simulink model "mfordmodel_v1"  (R2023a)
settings: Solver=ode45  StartTime=0.0  StopTime=10.0  RelTol=1e-3  EnableMultiTasking=on
undefined symbols (not defined in the file): ABV_RATIO_SW, AC_OFF_DLY, ACLOD, AUTO_TRNS_SW, BRAKE_DNDT_X, BZZRPM, BZZRPM_ALT, BZZTM, BZZTM_ALT, CMD_LITOFF, CMD_STABLE, CO_ST_ECT__A, COOL_BASE, DAS_BKDLY_A, DAS_CNT, DAS_CTDLY, DAS_LC_SW__A, DASCLP_5INH, DASCTL, DASMHYST, DASMPH, DEBYCP, DES_BASE, DPNEU_MUL, DSDRPM_DN_TC, DSDRPM_OFF, DSDRPM_UP_TC, EDF_DELAY, EDFHP, ETC_CL_TP, ETC_HP, GR_CM_CREEP, HCAM_ACT_CLP, HEDFHP, HEDFRPM, HICAM_PS, IAC_CAL_SW, IAC_ER_TM1, IAC_ER_TM2, IAC_ER_TM4, IAC_HI_LIM__A, IAC_ISFL_OBD, IAC_KAM_SW, IAC_LO_LIM__A, IAC_MON_TM, IAC_OT_REQ, IAC_RUN_TM, IAC_TP_OBD, IAC_TR_DAS, IAC_TST_DC, ID_DAS__A, ID_NOVS__A, IDVS_CH__A, IDVS_SL__A, IPSI_SW, IPSIDLY, IS_DRBASE__A, IS_DRBASE_A__A, IS_NUBASE__A, IS_NUBASE_A__A ... (+35)
libraries: simulink x2
(part 3 of 12)

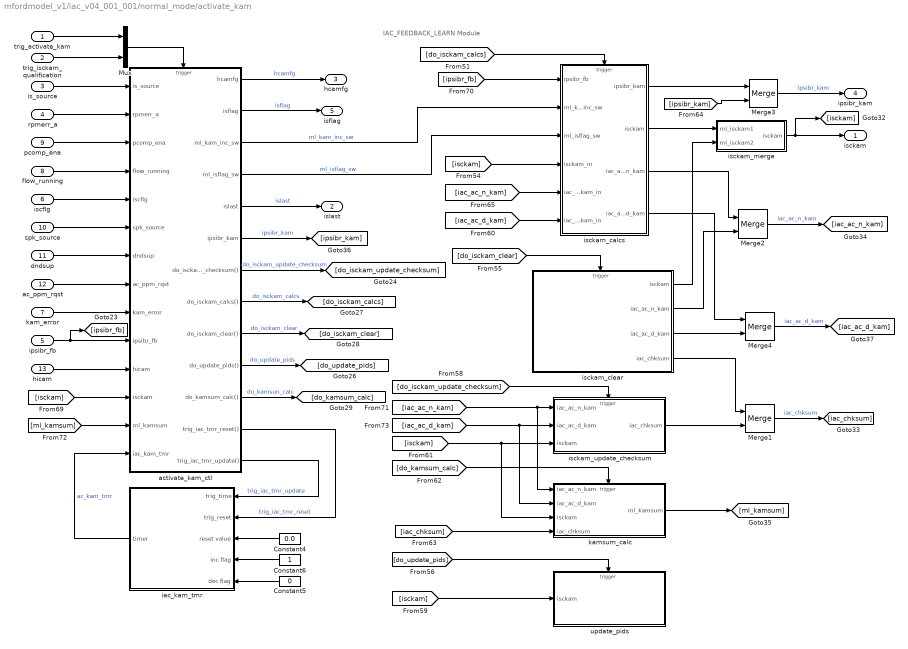
== system mfordmodel_v1/iac_v04_001_001/normal_mode/activate_kam ==
  note: IAC_FEEDBACK_LEARN Module
  trig_activate_kam : Inport
  trig_isckam_qualification : Inport  Port=2
  is_source : Inport  Port=3
  rpmerr_a : Inport  Port=4
  ipsibr_fb : Inport  Port=5
  iscflg : Inport  Port=6
  kam_error : Inport  Port=7
  flow_running : Inport  Port=8
  pcomp_ena : Inport  Port=9
  spk_source : Inport  Port=10
  dndsup : Inport  Port=11
  ac_ppm_rqst : Inport  Port=12
  hicam : Inport  Port=13
  Constant4 : Constant  Value=0.0
  Constant5 : Constant  Value=0
  Constant6 : Constant
  Merge{1..4} (4 alike) : Merge
  Mux : Mux  Inputs=2
  activate_kam_ctl : Stateflow chart  TreatAsAtomicUnit=on
  iac_kam_tmr : Subsystem  mask(TIMER){timer_name=iac_kam_tmr, init_value=0, clipped=off, tmin=, tmax=, unit_str=seconds}
      mask prompts: timer_name "Enter Timer Name"; init_value "initial TIMER value (in seconds)"; clipped "Clip timer?"; tmin "Minimum clip"; tmax "Maximum clip"; unit_str "Select timer units"
      mask help: Acts as a timer. Can count up, down, hold, or reset to zero. The required inputs are a timer function call, a reset function call, a reset value, an increment flag, and a decrement flag. Timer initial value, max and min clip values and timer name are selected below.
      mask init: same as mfordmodel_v1/iac_v04_001_001/normal_mode/activate_feedforward/ac_ppm_tmr
      mask Help:
      | <b><font size="+2">Input/Output Ports</font></b><br>
      | <p>
      | <b>Trig_timer:</b><br>
      | Connect a function call input to the 'trig_timer' port.  A function call passed through this port will activate the TIMER tool.  Activation updates the TIMER output.
      | <p>
      | <b>Trig_reset:</b><br>
      | Connect a function call input to the 'trig_reset' port.  A function call passed through this port will activate the TIMER tool.  Activation resets the TIMER output to the value passed to the 'reset_value' port.
      | <p>
      | <b>Reset_value:</b><br>
      | When 'trig_reset' is activated, the TIMER value will be reset to the real value passed to this input.
      | <p>
      | <b>Increment_flag and decrement_flag:</b><br>
      | If 'increment_flag' is 1 and 'decrement_flag' is 0, TIMER counts up.
      | If 'decrement_flag' is 1 and 'increment_flag' is 0, TIMER counts down.
      | If the flags are both 0 or both 1, TIMER holds its current value.
      | <p>
      | <b><font size="+2">Parameter Selection:</font></b>
      | <p>
      | <b>Initial TIMER Value:</b><br>
      | TIMER will begin at specified value.  Enter in seconds.
      mask TypeOptions unit_str: seconds | milliseconds
      mask Display:
      | plot( [0.3 0.45 0.55 0.7], [0.4 0.4 0.6 0.6])
      | plot( [ .475 .435 .415  .4 .4  .415 .435 .475  .525 .565 .585 .6 .6  ...
      | .585 .565 .525 .475], [.9  .885 .865  .825 .775 .735 .715  .7 .7 ...
      | .715 .735 .775 .825  .865 .885 .9 .9] )
      | plot( [.5 .5], [.89 .87])
      | plot( [.5 .5], [.71 .73])
      | plot( [.41 .43], [.8 .8])
      | plot( [.57 .59], [.8 .8])
      | plot( [.5 .5], [.8 .89])
      | plot( [.49 .5 .51], [.88 .89 .88] )
      | plot( [.5 .555], [.8 .825] )
      | plot( [.535 .555 .555], [.825 .825 .815])
      | text(0.35, 0.35, min_text)
      | text(0.6, 0.7,max_text)
      | text( 0.35, .95, timer_name)
  isckam_calcs : Subsystem  TreatAsAtomicUnit=on
  isckam_clear : Subsystem  TreatAsAtomicUnit=on  mask(isckam_clear){}
      mask help: TBD
      mask Display:
      | disp('
      | isckam0 = IAC_DR_START               \n
      | isckam1 = 0.0                                  \n
      | isckam2 = IAC_NU_START               \n
      | isckam3 = 0.0                                  \n
      | iac_ac_d_kam = IAC_AC_START       \n
      | iac_ac_n_kam = IAC_AC_START       \n
      | iac_chksum = ( isckam2 + isckam0 + \n
      |  iac_ac_d_kam + iac_ac_n_kam)         ' )
  isckam_merge : Subsystem  mask(vector_merge){}
      mask help: Merge the four elements of the "isckam" vector.
      mask Display: disp('Merge( isckam[i] )')
  isckam_update_checksum : Subsystem  TreatAsAtomicUnit=on  mask(isckam_update_checksum){}
      mask help: Computes and returns the checksum.
      mask Display:
      | disp('
      | iac_chksum = isckam[0] + \n
      |  isckam[2] +          \n
      | iac_ac_d_kam +  \n
      | iac_ac_n_ham     ')
  kamsum_calc : Subsystem  TreatAsAtomicUnit=on  mask(kam_sum_calc){}
      mask help: TBD
      mask Display:
      | fprintf(' ml_kamsum = ABS ( isckam[0] + \n
      | isckam[2] + iac_ac_n_kam + \n
      | iac_ac_d_kam - iac_chksum )')
  update_pids : Subsystem  TreatAsAtomicUnit=on  mask(update_pids){}
      mask help: Update isckam PIDS.
      mask Display:
      | disp ('Update the following PIDS:\n
      | J2190_0x0976 = isckam[0]\n
      | J2190_0x0977 = isckam[1]\n
      | J2190_0x0978 = isckam[2]\n
      | J2190_0x0979 = isckam[3]')
  isckam : Outport  InitialOutput=0
  islast : Outport  Port=2  InitialOutput=0
  hcamfg : Outport  Port=3  InitialOutput=0
  ipsibr_kam : Outport  Port=4  InitialOutput=0
  isflag : Outport  Port=5  InitialOutput=0
  wires:
  rpmerr_a/1 -> activate_kam_ctl/2(rpmerr_a)
  is_source/1 -> activate_kam_ctl/1(is_source)
  pcomp_ena/1 -> activate_kam_ctl/3(pcomp_ena)
  flow_running/1 -> activate_kam_ctl/4(flow_running)
  iscflg/1 -> activate_kam_ctl/5(iscflg)
  spk_source/1 -> activate_kam_ctl/6(spk_source)
  dndsup/1 -> activate_kam_ctl/7(dndsup)
  ac_ppm_rqst/1 -> activate_kam_ctl/8(ac_ppm_rqst)
  kam_error/1 -> activate_kam_ctl/9(kam_error)
  activate_kam_ctl/1(hcamfg) -> hcamfg/1  "hcamfg"
  activate_kam_ctl/5(islast) -> islast/1  "islast"
  [isckam] -> activate_kam_ctl/12(isckam)
  activate_kam_ctl/7(do_isckam_update_checksum()) -> [do_isckam_update_checksum]  "do_isckam_update_checksum"
  activate_kam_ctl/10(do_update_pids()) -> [do_update_pids]  "do_update_pids"
  activate_kam_ctl/12(trig_iac_tmr_reset()) -> iac_kam_tmr/2(trig_reset)  "trig_iac_tmr_reset"
  activate_kam_ctl/13(trig_iac_tmr_update()) -> iac_kam_tmr/1(trig_time)  "trig_iac_tmr_update"
  Constant5/1 -> iac_kam_tmr/5(dec flag)
  activate_kam_ctl/8(do_isckam_calcs()) -> [do_isckam_calcs]  "do_isckam_calcs"
  activate_kam_ctl/9(do_isckam_clear()) -> [do_isckam_clear]  "do_isckam_clear"
  hicam/1 -> activate_kam_ctl/11(hicam)
  trig_activate_kam/1 -> Mux/1
  Mux/1 -> activate_kam_ctl/Trigger
  trig_isckam_qualification/1 -> Mux/2
  activate_kam_ctl/11(do_kamsum_calc()) -> [do_kamsum_calc]  "do_kamsun_calc"
  Constant6/1 -> iac_kam_tmr/4(inc flag)
  Constant4/1 -> iac_kam_tmr/3(reset value)
  iac_kam_tmr/1(timer) -> activate_kam_ctl/14(iac_kam_tmr)  "ac_kam_tmr"
  [ml_kamsum] -> activate_kam_ctl/13(ml_kamsum)
  activate_kam_ctl/6(ipsibr_kam) -> [ipsibr_kam]  "ipsibr_kam"
  activate_kam_ctl/2(isflag) -> isflag/1  "isflag"
  isckam_clear/4(iac_chksum) -> Merge1/1
  [do_isckam_clear] -> isckam_clear/Trigger
  isckam_clear/1(isckam) -> isckam_merge/2(ml_isckam2)
  isckam_calcs/2(isckam) -> isckam_merge/1(ml_isckam1)
  isckam_calcs/3(iac_ac_n_kam) -> Merge2/1
  activate_kam_ctl/3(ml_kam_inc_sw) -> isckam_calcs/2(ml_kam_inc_sw)  "ml_kam_inc_sw"
  activate_kam_ctl/4(ml_isflag_sw) -> isckam_calcs/3(ml_isflag_sw)  "ml_isflag_sw"
  [do_isckam_calcs] -> isckam_calcs/Trigger
  [ipsibr_fb] -> isckam_calcs/1(ipsibr_fb)
  [isckam] -> isckam_calcs/4(isckam_in)
  [iac_ac_d_kam] -> isckam_calcs/6(iac_ac_d_kam_in)
  isckam_calcs/1(ipsibr_kam) -> Merge3/1
  [ipsibr_kam] -> Merge3/2
  Merge3/1 -> ipsibr_kam/1  "ipsibr_kam"
  isckam_calcs/4(iac_ac_d_kam) -> Merge4/1
  [iac_ac_n_kam] -> isckam_calcs/5(iac_ac_n_kam_in)
  isckam_clear/2(iac_ac_n_kam) -> Merge2/2
  isckam_clear/3(iac_ac_d_kam) -> Merge4/2
  isckam_merge/1(isckam) -> isckam/1, [isckam]
  [do_isckam_update_checksum] -> isckam_update_checksum/Trigger
  [isckam] -> update_pids/1(isckam)
  [do_update_pids] -> update_pids/Trigger
  isckam_update_checksum/1(iac_chksum) -> Merge1/2
  kamsum_calc/1(ml_kamsum) -> [ml_kamsum]
  [do_kamsum_calc] -> kamsum_calc/Trigger
  [iac_ac_n_kam] -> isckam_update_checksum/1(iac_ac_n_kam), kamsum_calc/1(iac_ac_n_kam)
  [isckam] -> isckam_update_checksum/3(isckam), kamsum_calc/3(isckam)
  [iac_chksum] -> kamsum_calc/4(iac_chksum)
  [iac_ac_d_kam] -> isckam_update_checksum/2(iac_ac_d_kam), kamsum_calc/2(iac_ac_d_kam)
  Merge2/1 -> [iac_ac_n_kam]  "iac_ac_n_kam"
  Merge1/1 -> [iac_chksum]  "iac_chksum"
  Merge4/1 -> [iac_ac_d_kam]  "iac_ac_d_kam"
  ipsibr_fb/1 -> [ipsibr_fb], activate_kam_ctl/10(ipsibr_fb)

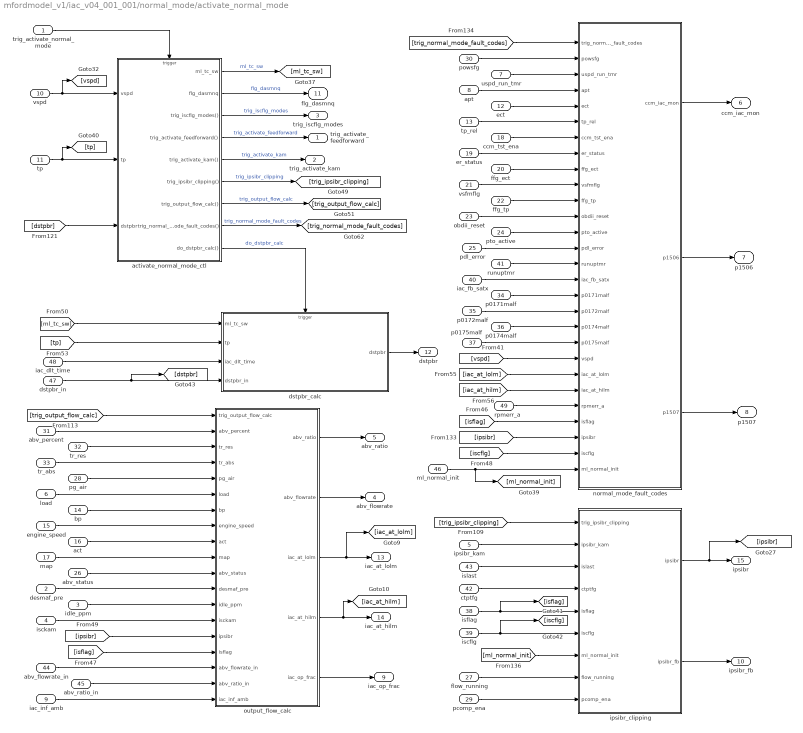
== system mfordmodel_v1/iac_v04_001_001/normal_mode/activate_normal_mode ==
  trig_activate_normal_mode : Inport
  desmaf_pre : Inport  Port=2
  idle_ppm : Inport  Port=3
  isckam : Inport  Port=4
  ipsibr_kam : Inport  Port=5
  load : Inport  Port=6
  uspd_run_tmr : Inport  Port=7
  apt : Inport  Port=8
  iac_inf_amb : Inport  Port=9
  vspd : Inport  Port=10
  tp : Inport  Port=11
  ect : Inport  Port=12
  tp_rel : Inport  Port=13
  bp : Inport  Port=14
  engine_speed : Inport  Port=15
  act : Inport  Port=16
  map : Inport  Port=17
  ccm_tst_ena : Inport  Port=18
  er_status : Inport  Port=19
  ffg_ect : Inport  Port=20
  vsfmflg : Inport  Port=21
  ffg_tp : Inport  Port=22
  obdii_reset : Inport  Port=23
  pto_active : Inport  Port=24
  pdl_error : Inport  Port=25
  abv_status : Inport  Port=26
  flow_running : Inport  Port=27
  pg_air : Inport  Port=28
  pcomp_ena : Inport  Port=29
  powsfg : Inport  Port=30
  abv_percent : Inport  Port=31
  tr_res : Inport  Port=32
  tr_abs : Inport  Port=33
  p0171malf : Inport  Port=34
  p0172malf : Inport  Port=35
  p0174malf : Inport  Port=36
  p0175malf : Inport  Port=37
  isflag : Inport  Port=38
  iscflg : Inport  Port=39
  iac_fb_satx : Inport  Port=40
  runuptmr : Inport  Port=41
  ctptfg : Inport  Port=42
  islast : Inport  Port=43
  abv_flowrate_in : Inport  Port=44
  abv_ratio_in : Inport  Port=45
  ml_normal_init : Inport  Port=46
  dstpbr_in : Inport  Port=47
  iac_dlt_time : Inport  Port=48
  rpmerr_a : Inport  Port=49
  activate_normal_mode_ctl : Stateflow chart  TreatAsAtomicUnit=on
  dstpbr_calc : Subsystem  TreatAsAtomicUnit=on  mask(dstpbr_calc){}
      mask help: TBD
      mask Display:
      | disp('\n
      | IF (ml_tc_sw == 1) THEN                                      \n
      | Tau = TCDASU                                              \n
      | ELSE IF (ml_tc_sw == 2) THEN                            \n
      | Tau = TCDASD                                              \n
      | ENDIF                                                                  \n
      | dstpbr = rolav_tc(dstpbr_in, tp, iac_dlt_time, Tau)     \n\n
      | ')
  ipsibr_clipping : Subsystem
  normal_mode_fault_codes : Subsystem
  output_flow_calc : Subsystem
  trig_activate_feedforward : Outport
  trig_activate_kam : Outport  Port=2
  trig_iscflg_modes : Outport  Port=3
  abv_flowrate : Outport  Port=4
  abv_ratio : Outport  Port=5
  ccm_iac_mon : Outport  Port=6
  p1506 : Outport  Port=7
  p1507 : Outport  Port=8
  iac_op_frac : Outport  Port=9
  ipsibr_fb : Outport  Port=10
  flg_dasmnq : Outport  Port=11
  dstpbr : Outport  Port=12
  iac_at_lolm : Outport  Port=13
  iac_at_hilm : Outport  Port=14
  ipsibr : Outport  Port=15
  wires:
  isflag/1 -> ipsibr_clipping/5(isflag), [isflag]
  iscflg/1 -> ipsibr_clipping/6(iscflg), [iscflg]
  pcomp_ena/1 -> ipsibr_clipping/9(pcomp_ena)
  flow_running/1 -> ipsibr_clipping/8(flow_running)
  ml_normal_init/1 -> normal_mode_fault_codes/28(ml_normal_init), [ml_normal_init]
  dstpbr_in/1 -> dstpbr_calc/4(dstpbr_in), [dstpbr]
  dstpbr_calc/1(dstpbr) -> dstpbr/1
  [trig_normal_mode_fault_codes] -> normal_mode_fault_codes/1(trig_normal_mode_fault_codes)
  [vspd] -> normal_mode_fault_codes/21(vspd)
  normal_mode_fault_codes/1(ccm_iac_mon) -> ccm_iac_mon/1
  normal_mode_fault_codes/2(p1506) -> p1506/1
  normal_mode_fault_codes/3(p1507) -> p1507/1
  pdl_error/1 -> normal_mode_fault_codes/14(pdl_error)
  apt/1 -> normal_mode_fault_codes/4(apt)
  uspd_run_tmr/1 -> normal_mode_fault_codes/3(uspd_run_tmr)
  ect/1 -> normal_mode_fault_codes/5(ect)
  tp_rel/1 -> normal_mode_fault_codes/6(tp_rel)
  [iscflg] -> normal_mode_fault_codes/27(iscflg)
  [isflag] -> normal_mode_fault_codes/25(isflag)
  rpmerr_a/1 -> normal_mode_fault_codes/24(rpmerr_a)
  ccm_tst_ena/1 -> normal_mode_fault_codes/7(ccm_tst_ena)
  er_status/1 -> normal_mode_fault_codes/8(er_status)
  ffg_ect/1 -> normal_mode_fault_codes/9(ffg_ect)
  vsfmflg/1 -> normal_mode_fault_codes/10(vsfmflg)
  ffg_tp/1 -> normal_mode_fault_codes/11(ffg_tp)
  obdii_reset/1 -> normal_mode_fault_codes/12(obdii_reset)
  pto_active/1 -> normal_mode_fault_codes/13(pto_active)
  iac_fb_satx/1 -> normal_mode_fault_codes/16(iac_fb_satx)
  runuptmr/1 -> normal_mode_fault_codes/15(runuptmr)
  p0171malf/1 -> normal_mode_fault_codes/17(p0171malf)
  p0172malf/1 -> normal_mode_fault_codes/18(p0172malf)
  p0174malf/1 -> normal_mode_fault_codes/19(p0174malf)
  p0175malf/1 -> normal_mode_fault_codes/20(p0175malf)
  [ipsibr] -> normal_mode_fault_codes/26(ipsibr)
  [iac_at_lolm] -> normal_mode_fault_codes/22(iac_at_lolm)
  [iac_at_hilm] -> normal_mode_fault_codes/23(iac_at_hilm)
  powsfg/1 -> normal_mode_fault_codes/2(powsfg)
  trig_activate_normal_mode/1 -> activate_normal_mode_ctl/Trigger
  activate_normal_mode_ctl/1(ml_tc_sw) -> [ml_tc_sw]  "ml_tc_sw"
  activate_normal_mode_ctl/2(flg_dasmnq) -> flg_dasmnq/1  "flg_dasmnq"
  [dstpbr] -> activate_normal_mode_ctl/3(dstpbr)
  vspd/1 -> activate_normal_mode_ctl/1(vspd), [vspd]
  tp/1 -> activate_normal_mode_ctl/2(tp), [tp]
  activate_normal_mode_ctl/9(do_dstpbr_calc()) -> dstpbr_calc/Trigger  "do_dstpbr_calc"
  ipsibr_clipping/2(ipsibr_fb) -> ipsibr_fb/1
  islast/1 -> ipsibr_clipping/3(islast)
  ctptfg/1 -> ipsibr_clipping/4(ctptfg)
  [trig_ipsibr_clipping] -> ipsibr_clipping/1(trig_ipsibr_clipping)
  ipsibr_kam/1 -> ipsibr_clipping/2(ipsibr_kam)
  [ml_normal_init] -> ipsibr_clipping/7(ml_normal_init)
  output_flow_calc/1(abv_ratio) -> abv_ratio/1
  output_flow_calc/2(abv_flowrate) -> abv_flowrate/1
  activate_normal_mode_ctl/3(trig_iscflg_modes()) -> trig_iscflg_modes/1  "trig_iscflg_modes"
  activate_normal_mode_ctl/6(trig_ipsibr_clipping()) -> [trig_ipsibr_clipping]  "trig_ipsibr_clipping"
  activate_normal_mode_ctl/7(trig_output_flow_calc()) -> [trig_output_flow_calc]  "trig_output_flow_calc"
  activate_normal_mode_ctl/8(trig_normal_mode_fault_codes()) -> [trig_normal_mode_fault_codes]  "trig_normal_mode_fault_codes"
  activate_normal_mode_ctl/4(trig_activate_feedforward()) -> trig_activate_feedforward/1  "trig_activate_feedforward"
  activate_normal_mode_ctl/5(trig_activate_kam()) -> trig_activate_kam/1  "trig_activate_kam"
  [trig_output_flow_calc] -> output_flow_calc/1(trig_output_flow_calc)
  [isflag] -> output_flow_calc/16(isflag)
  [ipsibr] -> output_flow_calc/15(ipsibr)
  desmaf_pre/1 -> output_flow_calc/12(desmaf_pre)
  idle_ppm/1 -> output_flow_calc/13(idle_ppm)
  isckam/1 -> output_flow_calc/14(isckam)
  load/1 -> output_flow_calc/6(load)
  bp/1 -> output_flow_calc/7(bp)
  engine_speed/1 -> output_flow_calc/8(engine_speed)
  act/1 -> output_flow_calc/9(act)
  map/1 -> output_flow_calc/10(map)
  abv_status/1 -> output_flow_calc/11(abv_status)
  pg_air/1 -> output_flow_calc/5(pg_air)
  abv_percent/1 -> output_flow_calc/2(abv_percent)
  tr_res/1 -> output_flow_calc/3(tr_res)
  tr_abs/1 -> output_flow_calc/4(tr_abs)
  abv_flowrate_in/1 -> output_flow_calc/17(abv_flowrate_in)
  abv_ratio_in/1 -> output_flow_calc/18(abv_ratio_in)
  iac_dlt_time/1 -> dstpbr_calc/3(iac_dlt_time)
  [ml_tc_sw] -> dstpbr_calc/1(ml_tc_sw)
  [tp] -> dstpbr_calc/2(tp)
  ipsibr_clipping/1(ipsibr) -> [ipsibr], ipsibr/1
  output_flow_calc/3(iac_at_lolm) -> [iac_at_lolm], iac_at_lolm/1
  output_flow_calc/5(iac_op_frac) -> iac_op_frac/1
  output_flow_calc/4(iac_at_hilm) -> [iac_at_hilm], iac_at_hilm/1
  iac_inf_amb/1 -> output_flow_calc/19(iac_inf_amb)

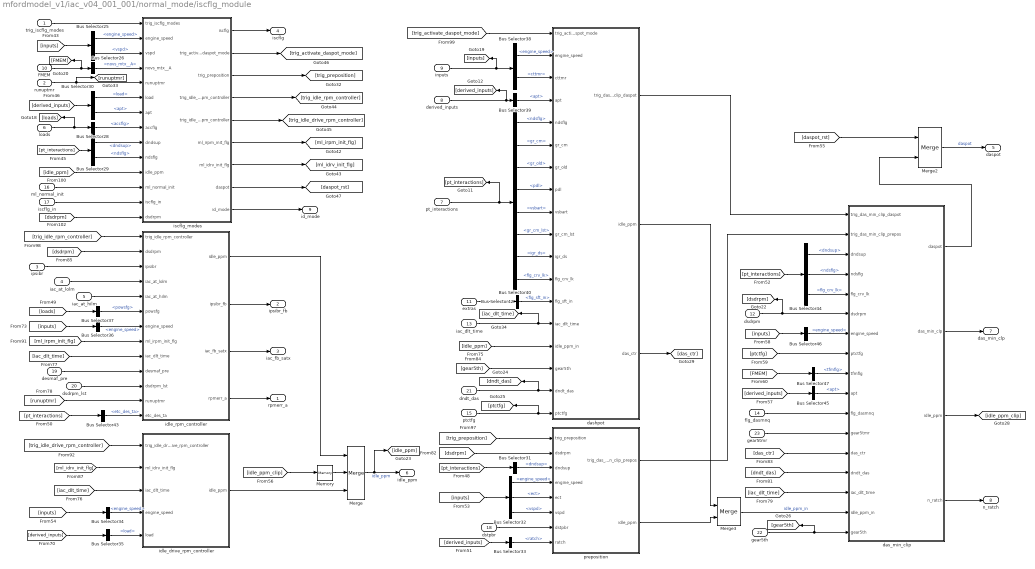
== system mfordmodel_v1/iac_v04_001_001/normal_mode/iscflg_module ==
  trig_iscflg_modes : Inport
  runuptmr : Inport  Port=2
  ipsibr : Inport  Port=3
  iac_at_lolm : Inport  Port=4
  iac_at_hilm : Inport  Port=5
  loads : Inport  Port=6
  pt_interactions : Inport  Port=7
  derived_inputs : Inport  Port=8
  inputs : Inport  Port=9
  FMEM : Inport  Port=10
  extras : Inport  Port=11
  dsdrpm : Inport  Port=12
  iac_dlt_time : Inport  Port=13
  flg_dasmnq : Inport  Port=14
  ptctfg : Inport  Port=15
  ml_normal_init : Inport  Port=16
  iscflg_in : Inport  Port=17
  dstpbr : Inport  Port=18
  desmaf_pre : Inport  Port=19
  dsdrpm_lst : Inport  Port=20
  dndt_das : Inport  Port=21
  gear5th : Inport  Port=22
  gear5tmr : Inport  Port=23
  Bus Selector25 : BusSelector  OutputSignals=engine_speed,vspd
  Bus Selector26 : BusSelector  OutputSignals=novs_mtx__A
  Bus Selector28 : BusSelector  OutputSignals=accflg
  Bus Selector29 : BusSelector  OutputSignals=dndsup,ndsflg
  Bus Selector30 : BusSelector  OutputSignals=load,apt
  Bus Selector31 : BusSelector  OutputSignals=dndsup
  Bus Selector32 : BusSelector  OutputSignals=engine_speed,ect,vspd
  Bus Selector33 : BusSelector  OutputSignals=ratch
  Bus Selector34 : BusSelector  OutputSignals=engine_speed
  Bus Selector35 : BusSelector  OutputSignals=load
  Bus Selector36 : BusSelector  OutputSignals=engine_speed
  Bus Selector37 : BusSelector  OutputSignals=powsfg
  Bus Selector38 : BusSelector  OutputSignals=engine_speed,cttmr
  Bus Selector39 : BusSelector  OutputSignals=apt
  Bus Selector40 : BusSelector  OutputSignals=ndsflg,gr_cm,gr_old,pdl,vsbart,gr_cm_lst,igr_ds,flg_crv_lk
  Bus Selector42 : BusSelector  OutputSignals=flg_sft_in
  Bus Selector43 : BusSelector  OutputSignals=etc_des_ta
  Bus Selector44 : BusSelector  OutputSignals=dndsup,ndsflg,flg_crv_lk
  Bus Selector45 : BusSelector  OutputSignals=apt
  Bus Selector46 : BusSelector  OutputSignals=engine_speed
  Bus Selector47 : BusSelector  OutputSignals=tfmflg
  Memory : Memory
  Merge : Merge  Inputs=3
  Merge2 : Merge
  Merge3 : Merge
  das_min_clip : Subsystem
  dashpot : Subsystem
  idle_drive_rpm_controller : Subsystem
  idle_rpm_controller : Subsystem
  iscflg_modes : Subsystem
  preposition : Subsystem
  rpmerr_a : Outport
  ipsibr_fb : Outport  Port=2
  iac_fb_satx : Outport  Port=3
  iscflg : Outport  Port=4
  daspot : Outport  Port=5
  idle_ppm : Outport  Port=6
  das_min_clp : Outport  Port=7
  n_ratch : Outport  Port=8
  id_mode : Outport  Port=9
  wires:
  iscflg_modes/9(id_mode) -> id_mode/1
  das_min_clip/4(n_ratch) -> n_ratch/1
  [daspot_rst] -> Merge2/1
  das_min_clip/1(daspot) -> Merge2/2
  Merge2/1 -> daspot/1  "daspot"
  FMEM/1 -> [FMEM], Bus Selector26/1
  inputs/1 -> Bus Selector38/1, [inputs]
  Bus Selector38/2 -> dashpot/3(cttmr)  "<cttmr>"
  pt_interactions/1 -> Bus Selector40/1, [pt_interactions]
  iac_dlt_time/1 -> [iac_dlt_time], dashpot/14(iac_dlt_time)
  [gear5th] -> dashpot/16(gear5th)
  [idle_ppm] -> dashpot/15(idle_ppm_in)
  extras/1 -> Bus Selector42/1
  derived_inputs/1 -> Bus Selector39/1, [derived_inputs]
  dashpot/3(das_ctr) -> [das_ctr]
  Bus Selector44/3 -> das_min_clip/5(flg_crv_lk)  "<flg_crv_lk>"
  [ptctfg] -> das_min_clip/8(ptctfg)
  Bus Selector47/1 -> das_min_clip/9(tfmflg)  "<tfmflg>"
  [FMEM] -> Bus Selector47/1
  [derived_inputs] -> Bus Selector45/1
  [inputs] -> Bus Selector46/1
  Bus Selector46/1 -> das_min_clip/7(engine_speed)  "<engine_speed>"
  dsdrpm/1 -> [dsdrpm], das_min_clip/6(dsdrpm)
  Bus Selector45/1 -> das_min_clip/10(apt)  "<apt>"
  ptctfg/1 -> dashpot/18(ptctfg), [ptctfg]
  dndt_das/1 -> [dndt_das], dashpot/17(dndt_das)
  Bus Selector42/1 -> dashpot/13(flg_sft_in)  "<flg_sft_in>"
  Bus Selector40/8 -> dashpot/12(flg_crv_lk)  "<flg_crv_lk>"
  Bus Selector40/7 -> dashpot/11(igr_ds)  "<igr_ds>"
  Bus Selector40/5 -> dashpot/9(vsbart)  "<vsbart>"
  Bus Selector40/1 -> dashpot/5(ndsflg)  "<ndsflg>"
  Bus Selector38/1 -> dashpot/2(engine_speed)  "<engine_speed>"
  Bus Selector39/1 -> dashpot/4(apt)  "<apt>"
  Bus Selector40/2 -> dashpot/6(gr_cm)  "<gr_cm>"
  Bus Selector40/4 -> dashpot/8(pdl)  "<pdl>"
  Bus Selector40/6 -> dashpot/10(gr_cm_lst)  "<gr_cm_lst>"
  Bus Selector40/3 -> dashpot/7(gr_old)  "<gr_old>"
  preposition/1(trig_das_min_clip_prepos) -> das_min_clip/2(trig_das_min_clip_prepos)
  preposition/2(idle_ppm) -> Merge3/2
  [trig_preposition] -> preposition/1(trig_preposition)
  [dsdrpm] -> preposition/2(dsdrpm)
  Bus Selector31/1 -> preposition/3(dndsup)  "<dndsup>"
  [pt_interactions] -> Bus Selector31/1
  [inputs] -> Bus Selector32/1
  Bus Selector32/1 -> preposition/4(engine_speed)  "<engine_speed>"
  Bus Selector32/2 -> preposition/5(ect)  "<ect>"
  Bus Selector32/3 -> preposition/6(vspd)  "<vspd>"
  [derived_inputs] -> Bus Selector33/1
  Bus Selector33/1 -> preposition/8(ratch)  "<ratch>"
  dstpbr/1 -> preposition/7(dstpbr)
  gear5th/1 -> [gear5th], das_min_clip/17(gear5th)
  Bus Selector44/2 -> das_min_clip/4(ndsflg)  "<ndsflg>"
  Bus Selector44/1 -> das_min_clip/3(dndsup)  "<dndsup>"
  [pt_interactions] -> Bus Selector44/1
  flg_dasmnq/1 -> das_min_clip/11(flg_dasmnq)
  gear5tmr/1 -> das_min_clip/12(gear5tmr)
  [das_ctr] -> das_min_clip/13(das_ctr)
  [dndt_das] -> das_min_clip/14(dndt_das)
  [iac_dlt_time] -> das_min_clip/15(iac_dlt_time)
  das_min_clip/2(das_min_clp) -> das_min_clp/1
  das_min_clip/3(idle_ppm) -> [idle_ppm_clip]
  [trig_activate_daspot_mode] -> dashpot/1(trig_activate_daspot_mode)
  dashpot/1(trig_das_min_clip_daspot) -> das_min_clip/1(trig_das_min_clip_daspot)
  Merge3/1 -> das_min_clip/16(idle_ppm_in)  "idle_ppm_in"
  dashpot/2(idle_ppm) -> Merge3/1
  [idle_ppm_clip] -> Memory/1
  idle_drive_rpm_controller/1(idle_ppm) -> Merge/3
  iscflg_modes/8(daspot) -> [daspot_rst]
  ipsibr/1 -> idle_rpm_controller/3(ipsibr)
  idle_rpm_controller/1(idle_ppm) -> Merge/1
  Merge/1 -> idle_ppm/1, [idle_ppm]  "idle_ppm"
  Bus Selector36/1 -> idle_rpm_controller/7(engine_speed)  "<engine_speed>"
  Bus Selector37/1 -> idle_rpm_controller/6(powsfg)  "<powsfg>"
  [loads] -> Bus Selector37/1
  [inputs] -> Bus Selector36/1
  [pt_interactions] -> Bus Selector43/1
  Bus Selector43/1 -> idle_rpm_controller/13(etc_des_ta)  "<etc_des_ta>"
  [inputs] -> Bus Selector34/1
  Bus Selector35/1 -> idle_drive_rpm_controller/5(load)  "<load>"
  [derived_inputs] -> Bus Selector35/1
  [trig_idle_drive_rpm_controller] -> idle_drive_rpm_controller/1(trig_idle_drive_rpm_controller)
  [iac_dlt_time] -> idle_drive_rpm_controller/3(iac_dlt_time)
  Bus Selector34/1 -> idle_drive_rpm_controller/4(engine_speed)  "<engine_speed>"
  [ml_idrv_init_flg] -> idle_drive_rpm_controller/2(ml_idrv_init_flg)
  [runuptmr] -> idle_rpm_controller/12(runuptmr)
  dsdrpm_lst/1 -> idle_rpm_controller/11(dsdrpm_lst)
  desmaf_pre/1 -> idle_rpm_controller/10(desmaf_pre)
  [iac_dlt_time] -> idle_rpm_controller/9(iac_dlt_time)
  [ml_irpm_init_flg] -> idle_rpm_controller/8(ml_irpm_init_flg)
  iac_at_hilm/1 -> idle_rpm_controller/5(iac_at_hilm)
  iac_at_lolm/1 -> idle_rpm_controller/4(iac_at_lolm)
  [dsdrpm] -> idle_rpm_controller/2(dsdrpm)
  idle_rpm_controller/2(ipsibr_fb) -> ipsibr_fb/1
  idle_rpm_controller/3(iac_fb_satx) -> iac_fb_satx/1
  idle_rpm_controller/4(rpmerr_a) -> rpmerr_a/1
  [trig_idle_rpm_controller] -> idle_rpm_controller/1(trig_idle_rpm_controller)
  runuptmr/1 -> [runuptmr], iscflg_modes/5(runuptmr)
  iscflg_modes/3(trig_preposition) -> [trig_preposition]
  iscflg_modes/6(ml_irpm_init_flg) -> [ml_irpm_init_flg]
  iscflg_modes/7(ml_idrv_init_flg) -> [ml_idrv_init_flg]
  iscflg_modes/4(trig_idle_rpm_controller) -> [trig_idle_rpm_controller]
  iscflg_modes/5(trig_idle_drive_rpm_controller) -> [trig_idle_drive_rpm_controller]
  iscflg_modes/2(trig_activate_daspot_mode) -> [trig_activate_daspot_mode]
  iscflg_modes/1(iscflg) -> iscflg/1
  trig_iscflg_modes/1 -> iscflg_modes/1(trig_iscflg_modes)
  [derived_inputs] -> Bus Selector30/1
  [idle_ppm] -> iscflg_modes/11(idle_ppm)
  [pt_interactions] -> Bus Selector29/1
  loads/1 -> Bus Selector28/1, [loads]
  ml_normal_init/1 -> iscflg_modes/12(ml_normal_init)
  iscflg_in/1 -> iscflg_modes/13(iscflg_in)
  Bus Selector25/2 -> iscflg_modes/3(vspd)  "<vspd>"
  Bus Selector25/1 -> iscflg_modes/2(engine_speed)  "<engine_speed>"
  Bus Selector26/1 -> iscflg_modes/4(novs_mtx__A)  "<novs_mtx__A>"
  [inputs] -> Bus Selector25/1
  Bus Selector29/1 -> iscflg_modes/9(dndsup)  "<dndsup>"
  Bus Selector28/1 -> iscflg_modes/8(accflg)  "<accflg>"
  Bus Selector30/1 -> iscflg_modes/6(load)  "<load>"
  Bus Selector30/2 -> iscflg_modes/7(apt)  "<apt>"
  Bus Selector29/2 -> iscflg_modes/10(ndsflg)  "<ndsflg>"
  [dsdrpm] -> iscflg_modes/14(dsdrpm)
  Memory/1 -> Merge/2

== system mfordmodel_v1/iac_v04_001_001/activate_desired_rpm/base_rpm_and_select_logic/dsdrpm_calc ==
  dsdrpm_tmp : Inport
  dsdrpm_tc_tmp : Inport  Port=2
  iac_dlt_time : Inport  Port=3
  do_dsdrpm_calc : TriggerPort  TriggerType=function-call  VariantControl=(inherit)
  Constant : Constant  Value=0
  ROLAV_TC_in_DT_in : Subsystem  mask(Rolling Average - Time Constant){}
      mask help: Rolling Average - Time Constant. This filter block is the first order approximation using a time constant. Inputs include the time constant, old_ave which is the previous average value, new_value which is the new filter to filter toward, and the delta_time which is elapsed time over which to perform the filter equation.
      mask Display: fprintf('ROLAV_TC');
  Unit Delay : UnitDelay  SampleTime=-1
  pid : Subsystem  mask(PID){pid_cat=J2190, pid_number=0x1135, bit=BIT_NONE}
      mask prompts: pid_cat "PID Category"; pid_number "PID Number (e.g., 0x0C or 0x1123)"
      mask help:
      | Generic PID - used for J1979 (modes 1,2) and J2190.
      |
      | PID number is either 2 (J1979) or 4 ( J2190) digits, preceeded by 0x.
      |
      | BIT is selected from a pop-up list.
      |
      | CTRL is either CTRL_NONE (default) or your control parameter which enables/disables reporting of the PID.
      mask TypeOptions pid_cat: J1979MODE1 | J1979MODE2 | J1979MODE6 | J2190
      mask TypeOptions bit: BIT_NONE | BIT_00 | BIT_01 | BIT_02 | BIT_03 | BIT_04 | BIT_05 | BIT_06 | BIT_07 | BIT_08 | BIT_09 | BIT_10 | BIT_11 | BIT_12 | BIT_13 | BIT_14 | BIT_15 | BIT_16 | BIT_17 | BIT_18 | BIT_19 | BIT_20 | BIT_21 | BIT_22 | BIT_23 | BIT_24 | BIT_25 | BIT_26 | BIT_27 | BIT_28 | BIT_29 | BIT_30 | BIT_31
      mask Display: fprintf('%s\n%s\n%s',pid_cat,pid_number,bit);
  dsdrpm : Outport
  dsdrpm_lst : Outport  Port=2
  wires:
  Unit Delay/1 -> dsdrpm_lst/1, ROLAV_TC_in_DT_in/3(old_ave)  "dsdrpm_lst"
  ROLAV_TC_in_DT_in/1(new_ave) -> Unit Delay/1, dsdrpm/1, pid/1(data)  "dsdrpm"
  dsdrpm_tmp/1 -> ROLAV_TC_in_DT_in/1(new_value)
  dsdrpm_tc_tmp/1 -> ROLAV_TC_in_DT_in/2(Tau)
  iac_dlt_time/1 -> ROLAV_TC_in_DT_in/4(delta_time)
  Constant/1 -> pid/2(ctrl)

== system mfordmodel_v1/iac_v04_001_001/activate_desired_rpm/base_rpm_and_select_logic/htr_core_rpm_calc ==
  ml_heater_core_calc_sw : Inport
  iac_inf_amb : Inport  Port=2
  do_heater_core_rpm_calc : TriggerPort  TriggerType=function-call  VariantControl=(inherit)
  Multiport Switch : MultiPortSwitch  Inputs=2
  lookup_2d : Subsystem  mask(2-D, piece-wise, linear interpolation){CAL_FUNC=FN_NUBASE_IA}
      mask prompts: CAL_FUNC "Calibration function name"
      mask help:
      | Performs piece-wise linear interpolation.
      |
      | Output is NOT extrapolated beyond the input range.  If the input value presented to the block lies outside the range specified in the block's parameter, then the value is treated as though it has the value of the nearest value in the range.
      mask init: same as mfordmodel_v1/iac_v04_001_001/activate_desired_rpm/rpm_calcs/lookup_2d
      mask Help:
      | Enter the name of the calibration function.
      | (e.g. EGM_VA_ECT_MULT)
      mask Display:
      | fprintf('%s',CAL_FUNC);
      | plot(calfunc.X,calfunc.Y,max_x*1.05,max_y*1.05,min_x,min_y);
  lookup_2d1 : Subsystem  mask(2-D, piece-wise, linear interpolation){CAL_FUNC=FN_DRBASE_IA}
      mask prompts: CAL_FUNC "Calibration function name"
      mask help:
      | Performs piece-wise linear interpolation.
      |
      | Output is NOT extrapolated beyond the input range.  If the input value presented to the block lies outside the range specified in the block's parameter, then the value is treated as though it has the value of the nearest value in the range.
      mask init: same as mfordmodel_v1/iac_v04_001_001/activate_desired_rpm/rpm_calcs/lookup_2d
      mask Help:
      | Enter the name of the calibration function.
      | (e.g. EGM_VA_ECT_MULT)
      mask Display:
      | fprintf('%s',CAL_FUNC);
      | plot(calfunc.X,calfunc.Y,max_x*1.05,max_y*1.05,min_x,min_y);
  is_heater_core_rpm_tmp : Outport
  wires:
  ml_heater_core_calc_sw/1 -> Multiport Switch/1
  iac_inf_amb/1 -> lookup_2d1/1(In1), lookup_2d/1(In1)
  lookup_2d/1(Out1) -> Multiport Switch/2
  lookup_2d1/1(Out1) -> Multiport Switch/3
  Multiport Switch/1 -> is_heater_core_rpm_tmp/1  "is_heater_core_rpm_tmp"

== system mfordmodel_v1/iac_v04_001_001/activate_desired_rpm/hicam_rpm_request/fox_calcs ==
  act : Inport
  acstrt : Inport  Port=2
  tcstrt : Inport  Port=3
  ect : Inport  Port=4
  do_fox_calcs : TriggerPort  TriggerType=function-call  VariantControl=(inherit)
  CONSTANT : Subsystem  mask(Constant){constant=HCAM_ACT_CLP}
      mask help: Constant Block. Will dispaly constant name and value on the icon of the block
      mask init:
      | if isletter(constant(1))
      |   const = evalin('base',constant);
      |   name = constant;
      | else
      |   const = str2num(constant);
      |   name = 'CONST';
      | end;
      mask Display: fprintf('%s = %.4f',name,const);
  MinMax : MinMax  Inputs=2  InputSameDT=on  SaturateOnIntegerOverflow=on
  lookup_2d : Subsystem  mask(2-D, piece-wise, linear interpolation){CAL_FUNC=FN825B}
      mask prompts: CAL_FUNC "Calibration function name"
      mask help:
      | Performs piece-wise linear interpolation.
      |
      | Output is NOT extrapolated beyond the input range.  If the input value presented to the block lies outside the range specified in the block's parameter, then the value is treated as though it has the value of the nearest value in the range.
      mask init: same as mfordmodel_v1/iac_v04_001_001/activate_desired_rpm/rpm_calcs/lookup_2d
      mask Help:
      | Enter the name of the calibration function.
      | (e.g. EGM_VA_ECT_MULT)
      mask Display:
      | fprintf('%s',CAL_FUNC);
      | plot(calfunc.X,calfunc.Y,max_x*1.05,max_y*1.05,min_x,min_y);
  lookup_2d1 : Subsystem  mask(2-D, piece-wise, linear interpolation){CAL_FUNC=FN803A}
      mask prompts: CAL_FUNC "Calibration function name"
      mask help:
      | Performs piece-wise linear interpolation.
      |
      | Output is NOT extrapolated beyond the input range.  If the input value presented to the block lies outside the range specified in the block's parameter, then the value is treated as though it has the value of the nearest value in the range.
      mask init: same as mfordmodel_v1/iac_v04_001_001/activate_desired_rpm/rpm_calcs/lookup_2d
      mask Help:
      | Enter the name of the calibration function.
      | (e.g. EGM_VA_ECT_MULT)
      mask Display:
      | fprintf('%s',CAL_FUNC);
      | plot(calfunc.X,calfunc.Y,max_x*1.05,max_y*1.05,min_x,min_y);
  lookup_2d2 : Subsystem  mask(2-D, piece-wise, linear interpolation){CAL_FUNC=FN826A}
      mask prompts: CAL_FUNC "Calibration function name"
      mask help:
      | Performs piece-wise linear interpolation.
      |
      | Output is NOT extrapolated beyond the input range.  If the input value presented to the block lies outside the range specified in the block's parameter, then the value is treated as though it has the value of the nearest value in the range.
      mask init: same as mfordmodel_v1/iac_v04_001_001/activate_desired_rpm/rpm_calcs/lookup_2d
      mask Help:
      | Enter the name of the calibration function.
      | (e.g. EGM_VA_ECT_MULT)
      mask Display:
      | fprintf('%s',CAL_FUNC);
      | plot(calfunc.X,calfunc.Y,max_x*1.05,max_y*1.05,min_x,min_y);
  lookup_2d3 : Subsystem  mask(2-D, piece-wise, linear interpolation){CAL_FUNC=FN826B}
      mask prompts: CAL_FUNC "Calibration function name"
      mask help:
      | Performs piece-wise linear interpolation.
      |
      | Output is NOT extrapolated beyond the input range.  If the input value presented to the block lies outside the range specified in the block's parameter, then the value is treated as though it has the value of the nearest value in the range.
      mask init: same as mfordmodel_v1/iac_v04_001_001/activate_desired_rpm/rpm_calcs/lookup_2d
      mask Help:
      | Enter the name of the calibration function.
      | (e.g. EGM_VA_ECT_MULT)
      mask Display:
      | fprintf('%s',CAL_FUNC);
      | plot(calfunc.X,calfunc.Y,max_x*1.05,max_y*1.05,min_x,min_y);
  lookup_2d4 : Subsystem  mask(2-D, piece-wise, linear interpolation){CAL_FUNC=FN825A}
      mask prompts: CAL_FUNC "Calibration function name"
      mask help:
      | Performs piece-wise linear interpolation.
      |
      | Output is NOT extrapolated beyond the input range.  If the input value presented to the block lies outside the range specified in the block's parameter, then the value is treated as though it has the value of the nearest value in the range.
      mask init: same as mfordmodel_v1/iac_v04_001_001/activate_desired_rpm/rpm_calcs/lookup_2d
      mask Help:
      | Enter the name of the calibration function.
      | (e.g. EGM_VA_ECT_MULT)
      mask Display:
      | fprintf('%s',CAL_FUNC);
      | plot(calfunc.X,calfunc.Y,max_x*1.05,max_y*1.05,min_x,min_y);
  lookup_2d5 : Subsystem  mask(2-D, piece-wise, linear interpolation){CAL_FUNC=FN825A_ALT}
      mask prompts: CAL_FUNC "Calibration function name"
      mask help:
      | Performs piece-wise linear interpolation.
      |
      | Output is NOT extrapolated beyond the input range.  If the input value presented to the block lies outside the range specified in the block's parameter, then the value is treated as though it has the value of the nearest value in the range.
      mask init: same as mfordmodel_v1/iac_v04_001_001/activate_desired_rpm/rpm_calcs/lookup_2d
      mask Help:
      | Enter the name of the calibration function.
      | (e.g. EGM_VA_ECT_MULT)
      mask Display:
      | fprintf('%s',CAL_FUNC);
      | plot(calfunc.X,calfunc.Y,max_x*1.05,max_y*1.05,min_x,min_y);
  ml_fn825b : Outport
  ml_fn803a : Outport  Port=2
  ml_fn826a : Outport  Port=3
  ml_fn826b : Outport  Port=4
  ml_fn825a : Outport  Port=5
  ml_fn825a_alt : Outport  Port=6
  ml_isadd_min : Outport  Port=7
  wires:
  ect/1 -> lookup_2d4/1(In1), lookup_2d5/1(In1)
  lookup_2d5/1(Out1) -> ml_fn825a_alt/1  "ml_fn825a_alt"
  lookup_2d4/1(Out1) -> ml_fn825a/1  "ml_fn825a"
  act/1 -> lookup_2d3/1(In1), lookup_2d/1(In1)
  lookup_2d3/1(Out1) -> ml_fn826b/1  "ml_fn826b"
  lookup_2d2/1(Out1) -> ml_fn826a/1  "ml_fn826a"
  tcstrt/1 -> lookup_2d2/1(In1)
  lookup_2d1/1(Out1) -> ml_fn803a/1  "ml_fn803a"
  acstrt/1 -> lookup_2d1/1(In1)
  lookup_2d/1(Out1) -> ml_fn825b/1, MinMax/2  "ml_fn825b"
  CONSTANT/1(Out) -> MinMax/1
  MinMax/1 -> ml_isadd_min/1  "ml_isadd_min"

== system mfordmodel_v1/iac_v04_001_001/activate_desired_rpm/hicam_rpm_request/hicam_calc ==
  isadd_act_tmp : Inport
  isadd_ect_tmp : Inport  Port=2
  isadd_st_ect_tmp : Inport  Port=3
  isadd_st_act_tmp : Inport  Port=4
  isadd_buzz_tmp : Inport  Port=5
  ml_isadd_sw : Inport  Port=6
  ml_isadd_ext : Inport  Port=7
  do_hicam_calc : TriggerPort  TriggerType=function-call  VariantControl=(inherit)
  CONSTANT : Subsystem  mask(Constant){constant=IS_CMD_ADD}
      mask help: Constant Block. Will dispaly constant name and value on the icon of the block
      mask init:
      | if isletter(constant(1))
      |   const = evalin('base',constant);
      |   name = constant;
      | else
      |   const = str2num(constant);
      |   name = 'CONST';
      | end;
      mask Display: fprintf('%s = %.4f',name,const);
  Constant : Constant  Value=0.0
  Multiport Switch : MultiPortSwitch
  Sum : Sum  Inputs=++++++  InputSameDT=on  SaturateOnIntegerOverflow=on  OutDataTypeStr=Inherit: Same as first input
  hicam : Outport
  isadd_ext__A : Outport  Port=2
  wires:
  isadd_buzz_tmp/1 -> Sum/5
  isadd_st_act_tmp/1 -> Sum/4
  isadd_st_ect_tmp/1 -> Sum/3
  isadd_ect_tmp/1 -> Sum/2
  isadd_act_tmp/1 -> Sum/1
  Sum/1 -> hicam/1  "hicam"
  Multiport Switch/1 -> Sum/6, isadd_ext__A/1  "isadd_ext__A"
  ml_isadd_sw/1 -> Multiport Switch/1
  CONSTANT/1(Out) -> Multiport Switch/2
  ml_isadd_ext/1 -> Multiport Switch/3
  Constant/1 -> Multiport Switch/4

== system mfordmodel_v1/iac_v04_001_001/activate_desired_rpm/hicam_rpm_request/isadd_ramp ==
  ml_ramp_sw : Inport
  isadd_ext__A : Inport  Port=2
  iac_dlt_time : Inport  Port=3
  do_isadd_ramp : TriggerPort  TriggerType=function-call  VariantControl=(inherit)
  CONSTANT : Subsystem  mask(Constant){constant=IS_CMD_ADD}
      mask help: Constant Block. Will dispaly constant name and value on the icon of the block
      mask init:
      | if isletter(constant(1))
      |   const = evalin('base',constant);
      |   name = constant;
      | else
      |   const = str2num(constant);
      |   name = 'CONST';
      | end;
      mask Display: fprintf('%s = %.4f',name,const);
  Constant : Constant  Value=0.0
  Constant1 : Constant  Value=60
  Constant2 : Constant  Value=30
  Multiport Switch : MultiPortSwitch  Inputs=2
  Multiport Switch1 : MultiPortSwitch  Inputs=2
  ROLAV_TC_in_DT_in : Subsystem  mask(Rolling Average - Time Constant){}
      mask help: Rolling Average - Time Constant. This filter block is the first order approximation using a time constant. Inputs include the time constant, old_ave which is the previous average value, new_value which is the new filter to filter toward, and the delta_time which is elapsed time over which to perform the filter equation.
      mask Display: fprintf('ROLAV_TC');
  ml_isadd_ext : Outport
  wires:
  Multiport Switch/1 -> ROLAV_TC_in_DT_in/1(new_value)
  Multiport Switch1/1 -> ROLAV_TC_in_DT_in/2(Tau)
  isadd_ext__A/1 -> ROLAV_TC_in_DT_in/3(old_ave)
  Constant1/1 -> Multiport Switch1/2
  Constant2/1 -> Multiport Switch1/3
  ROLAV_TC_in_DT_in/1(new_ave) -> ml_isadd_ext/1  "ml_isadd_ext"
  iac_dlt_time/1 -> ROLAV_TC_in_DT_in/4(delta_time)
  ml_ramp_sw/1 -> Multiport Switch/1, Multiport Switch1/1
  CONSTANT/1(Out) -> Multiport Switch/2
  Constant/1 -> Multiport Switch/3

== system mfordmodel_v1/iac_v04_001_001/activate_desired_rpm/inf_amb_calc/ROLAV_TC_DT_in ==
  note: Using the first two terms of the series expansion:
      |
      |                     x                     x2
      |                                e   =  1  +  x  +  --  + ......
      |                                           2!
      |
      |       Simplifying, the exponential "f" becomes:
      |
      |                  - (FK_TMR/TC)              1
      |           f  =  1  -  e                    =  1  -  -------------  =  . . .
      |                                                    (FK_TMR/TC)
      |                           e
      |
      |                              1                      1
      |          f  =  1  -  ---------------------------------  =    ------------------- .
      |                                  1 + (FK_TMR / TC)       1 + (TC / FK_TMR)
  note: - (FK_TMR/TC)
      |                                    f  =  1  -  e
      |
      |       Where "f" is called the filter constant in the difference equation:
      |
      |                    new_average = f * new_value + (1 - f) * old_average
  note: new_average = [ (sample_interval)/(sample_interval + time_constant) ] * (new_value - old_ave) + old_ave
  new_value : Inport
  old_ave : Inport  Port=2
  delta_time : Inport  Port=3
  Elementary Math : Math  Operator=reciprocal  SignedPower=on
  Product : Product  Inputs=3  InputSameDT=on  RndMeth=Zero  SaturateOnIntegerOverflow=on  OutDataTypeStr=Inherit: Same as first input
  Sum : Sum  Inputs=-+  InputSameDT=on  SaturateOnIntegerOverflow=on  OutDataTypeStr=Inherit: Same as first input
  Sum1 : Sum  InputSameDT=on  SaturateOnIntegerOverflow=on  OutDataTypeStr=Inherit: Same as first input
  Sum2 : Sum  InputSameDT=on  SaturateOnIntegerOverflow=on  OutDataTypeStr=Inherit: Same as first input
  Time Constant : Constant  Value=tc
  new_ave : Outport
  wires:
  Time Constant/1 -> Sum1/2
  Sum2/1 -> new_ave/1
  old_ave/1 -> Sum2/1, Sum/1
  Product/1 -> Sum2/2
  Sum/1 -> Product/1
  Elementary Math/1 -> Product/3
  Sum1/1 -> Elementary Math/1
  new_value/1 -> Sum/2
  delta_time/1 -> Product/2, Sum1/1

== system mfordmodel_v1/iac_v04_001_001/activate_desired_rpm/rpm_calcs/  4 ==
  Constant : Constant  Value=const
  Out : Outport
  wires:
  Constant/1 -> Out/1

== system mfordmodel_v1/iac_v04_001_001/activate_desired_rpm/rpm_calcs/  5 ==
  Constant : Constant  Value=const
  Out : Outport
  wires:
  Constant/1 -> Out/1

== system mfordmodel_v1/iac_v04_001_001/activate_desired_rpm/rpm_calcs/lookup_2d ==
  In1 : Inport
  Look-Up Table1 : Lookup  InputValues=calfunc.X  Table=calfunc.Y
  Saturation1 : Saturate  UpperLimit=max_x  LowerLimit=min_x
  Out1 : Outport
  wires:
  In1/1 -> Saturation1/1
  Saturation1/1 -> Look-Up Table1/1
  Look-Up Table1/1 -> Out1/1

== system mfordmodel_v1/iac_v04_001_001/activate_desired_rpm/rpm_calcs/lookup_2d1 ==
  In1 : Inport
  Look-Up Table1 : Lookup  InputValues=calfunc.X  Table=calfunc.Y
  Saturation1 : Saturate  UpperLimit=max_x  LowerLimit=min_x
  Out1 : Outport
  wires:
  In1/1 -> Saturation1/1
  Saturation1/1 -> Look-Up Table1/1
  Look-Up Table1/1 -> Out1/1

== system mfordmodel_v1/iac_v04_001_001/activate_desired_rpm/rpm_calcs/lookup_2d2 ==
  In1 : Inport
  Look-Up Table1 : Lookup  InputValues=calfunc.X  Table=calfunc.Y
  Saturation1 : Saturate  UpperLimit=max_x  LowerLimit=min_x
  Out1 : Outport
  wires:
  In1/1 -> Saturation1/1
  Saturation1/1 -> Look-Up Table1/1
  Look-Up Table1/1 -> Out1/1

== system mfordmodel_v1/iac_v04_001_001/activate_desired_rpm/rpm_calcs/lookup_2d3 ==
  In1 : Inport
  Look-Up Table1 : Lookup  InputValues=calfunc.X  Table=calfunc.Y
  Saturation1 : Saturate  UpperLimit=max_x  LowerLimit=min_x
  Out1 : Outport
  wires:
  In1/1 -> Saturation1/1
  Saturation1/1 -> Look-Up Table1/1
  Look-Up Table1/1 -> Out1/1

== system mfordmodel_v1/iac_v04_001_001/activate_desired_rpm/rpm_calcs/lookup_2d4 ==
  In1 : Inport
  Look-Up Table1 : Lookup  InputValues=calfunc.X  Table=calfunc.Y
  Saturation1 : Saturate  UpperLimit=max_x  LowerLimit=min_x
  Out1 : Outport
  wires:
  In1/1 -> Saturation1/1
  Saturation1/1 -> Look-Up Table1/1
  Look-Up Table1/1 -> Out1/1

== system mfordmodel_v1/iac_v04_001_001/iac_executive/fault_code_setting/TIMER_DT_in ==
  note: timer14/TIMER
  note: Timer Control calls functions within the Time Calculator
      | after using the flags 'increment_flag' and 'decrement_flag'
      | to determine the direction of the timer.
  trig_time : Inport
  trig_reset : Inport  Port=2
  reset value : Inport  Port=3
  inc flag : Inport  Port=4
  dec flag : Inport  Port=5
  delta time : Inport  Port=6
  Event Triggers : Mux  Inputs=2
  Time Calculator : Subsystem
  Timer Control : Stateflow chart  TreatAsAtomicUnit=on
  timer : Outport
  wires:
  inc flag/1 -> Timer Control/1(incr_flag)  "increment_flag"
  dec flag/1 -> Timer Control/2(decr_flag)  "decrement_flag"
  Timer Control/4(do_timer()) -> Time Calculator/4(do_timer)  "do_timer"
  Timer Control/3(do_delta_time()) -> Time Calculator/3(do_delta_time)  "do_delta_time"
  Timer Control/2(reset_flag) -> Time Calculator/2(reset_val)  "reset_flag"
  Timer Control/1(count_direction) -> Time Calculator/1(count_direction)  "count_direction"
  Time Calculator/1(timer) -> timer/1  "timer"
  Event Triggers/1 -> Timer Control/Trigger
  trig_time/1 -> Event Triggers/1  "trig_timer"
  trig_reset/1 -> Event Triggers/2  "trig_reset"
  reset value/1 -> Time Calculator/5(reset_value)  "reset_value"
  delta time/1 -> Time Calculator/6(delta time)  "delta_time"

== system mfordmodel_v1/iac_v04_001_001/iac_executive/fault_code_setting/type1_fault_code ==
  trig_malfunction : Inport
  trig_clear_malf : Inport  Port=2
  Ground{,1..3} (4 alike) : Ground
  Mux : Mux  Inputs=2
  Mux1 : Mux  Inputs=5
  fault code_ctl : Stateflow chart  TreatAsAtomicUnit=on
  pxxxx : Outport
  wires:
  Ground1/1 -> Mux1/2  "pxxxstate"
  Ground2/1 -> Mux1/3  "pxxxmil_on"
  Ground3/1 -> Mux1/4  "pxxxfault"
  Ground/1 -> Mux1/1  "pxxxcnt"
  fault code_ctl/1(pxxxmalf) -> Mux1/5  "pxxxmalf"
  Mux1/1 -> pxxxx/1
  Mux/1 -> fault code_ctl/Trigger
  trig_clear_malf/1 -> Mux/2
  trig_malfunction/1 -> Mux/1

== system mfordmodel_v1/iac_v04_001_001/iac_executive/misc_calcs/TIMER_DT_in ==
  note: timer14/TIMER
  note: Timer Control calls functions within the Time Calculator
      | after using the flags 'increment_flag' and 'decrement_flag'
      | to determine the direction of the timer.
  trig_time : Inport
  trig_reset : Inport  Port=2
  reset value : Inport  Port=3
  inc flag : Inport  Port=4
  dec flag : Inport  Port=5
  delta time : Inport  Port=6
  Event Triggers : Mux  Inputs=2
  Time Calculator : Subsystem
  Timer Control : Stateflow chart  TreatAsAtomicUnit=on
  timer : Outport
  wires:
  inc flag/1 -> Timer Control/1(incr_flag)  "increment_flag"
  dec flag/1 -> Timer Control/2(decr_flag)  "decrement_flag"
  Timer Control/4(do_timer()) -> Time Calculator/4(do_timer)  "do_timer"
  Timer Control/3(do_delta_time()) -> Time Calculator/3(do_delta_time)  "do_delta_time"
  Timer Control/2(reset_flag) -> Time Calculator/2(reset_val)  "reset_flag"
  Timer Control/1(count_direction) -> Time Calculator/1(count_direction)  "count_direction"
  Time Calculator/1(timer) -> timer/1  "timer"
  Event Triggers/1 -> Timer Control/Trigger
  trig_time/1 -> Event Triggers/1  "trig_timer"
  trig_reset/1 -> Event Triggers/2  "trig_reset"
  reset value/1 -> Time Calculator/5(reset_value)  "reset_value"
  delta time/1 -> Time Calculator/6(delta time)  "delta_time"

== system mfordmodel_v1/iac_v04_001_001/iac_executive/misc_calcs/dndt_calc ==
  ml_dndt_sw : Inport
  dndti : Inport  Port=2
  iac_dlt_time : Inport  Port=3
  do_dndt_calc : TriggerPort  TriggerType=function-call  VariantControl=(inherit)
  Constant : Constant  Value=0.0
  Multiport Switch : MultiPortSwitch  Inputs=2
  ROLAV_TC_DT_in : Subsystem  mask(Rolling Average - Time Constant){TAU=TCNDT_DAS}
      mask prompts: TAU "Time Constant"
      mask help: Rolling Average - Time Constant. This filter block is the first order approximation using a time constant. Inputs include the time constant (entered through this dialogue), old_ave which is the previous average value, new_value which is the new filter to filter toward, and the delta_time which is elapsed time over which to perform the filter equation.
      mask init:
      | if isletter(TAU(1))
      |   tc = evalin('base',TAU);
      |   name = TAU;
      | else
      |   tc = str2num(TAU);
      |   name = 'TC';
      | end;
      mask Display: fprintf('%s = %.4f',name,tc);
  Unit Delay : UnitDelay  SampleTime=-1
  dndt_das : Outport
  wires:
  ml_dndt_sw/1 -> Multiport Switch/1
  Multiport Switch/1 -> Unit Delay/1, dndt_das/1  "dndt_das"
  Constant/1 -> Multiport Switch/2
  ROLAV_TC_DT_in/1(new_ave) -> Multiport Switch/3
  iac_dlt_time/1 -> ROLAV_TC_DT_in/3(delta_time)
  Unit Delay/1 -> ROLAV_TC_DT_in/2(old_ave)
  dndti/1 -> ROLAV_TC_DT_in/1(new_value)

== system mfordmodel_v1/iac_v04_001_001/iac_executive/misc_calcs/osc_response_triggered ==
  note: For now, stub Output State Control Response logic
  do_osc_response : TriggerPort  TriggerType=function-call  VariantControl=(inherit)

== system mfordmodel_v1/iac_v04_001_001/iac_executive/mode_control/crank_mode ==
  trig_crank_mode : Inport
  tcstrt : Inport  Port=2
  tslpip : Inport  Port=3
  ratch : Inport  Port=4
  crank_calcs : Subsystem  TreatAsAtomicUnit=on  mask(crank_calcs){}
      mask help: TBD
      mask Display:
      | fprintf(' IF (ml_flow_sel_sw == 1) THEN          \n
      | abv_flowrate =                   \n
      |  fox(FNCRANK_PPM, tcstrt)\n
      | ELSE IF (ml_flow_sel_sw == 2) THEN\n
      | abv_flowrate = 0.0              \n
      | ENDIF                                                \n
      | abv_ratio = 0                                 \n
      | hcamfg = 1                                    \n
      | iscflg = 0                                       \n
      | dstpbr = ratch                                 ')
  crank_mode_ctl : Stateflow chart  TreatAsAtomicUnit=on
  abv_flowrate : Outport
  abv_ratio : Outport  Port=2
  hcamfg : Outport  Port=3
  iscflg : Outport  Port=4
  dstpbr : Outport  Port=5
  wires:
  ratch/1 -> crank_calcs/3(ratch)
  crank_calcs/5(dstpbr) -> dstpbr/1
  crank_calcs/4(iscflg) -> iscflg/1
  crank_calcs/3(hcamfg) -> hcamfg/1
  crank_mode_ctl/1(ml_flow_sel_sw) -> crank_calcs/1(ml_flow_sel_sw)  "ml_flow_sel_sw"
  tcstrt/1 -> crank_calcs/2(tcstrt)
  trig_crank_mode/1 -> crank_mode_ctl/Trigger
  crank_mode_ctl/2(do_crank_calcs()) -> crank_calcs/Trigger  "do_crank_calcs"
  crank_calcs/1(abv_ratio) -> abv_ratio/1
  crank_calcs/2(abv_flowrate) -> abv_flowrate/1
  tslpip/1 -> crank_mode_ctl/1(tslpip)
